simulink model "MASS"  (R2018b)
settings: Solver=VariableStepAuto  StartTime=0.0  StopTime=10.0  RelTol=1e-3
values from neighbouring files (symbols this model uses):
  B = magic(4)    [exp13003.m]    (also in lab13003.m; lab1a3003.m = 2.5; lab2a3003.m = 2.5)
  F = 8    [lab1a3003.m]    (also in lab2a3003.m)
  K = 16    [lab1a3003.m]    (also in lab2a3003.m)
  M = 2    [lab1a3003.m]    (also in lab2a3003.m)
  x0 = 4    [lab1a3003.m]    (also in lab2a3003.m)
settings Model: Creator=student  LastModifiedBy=student

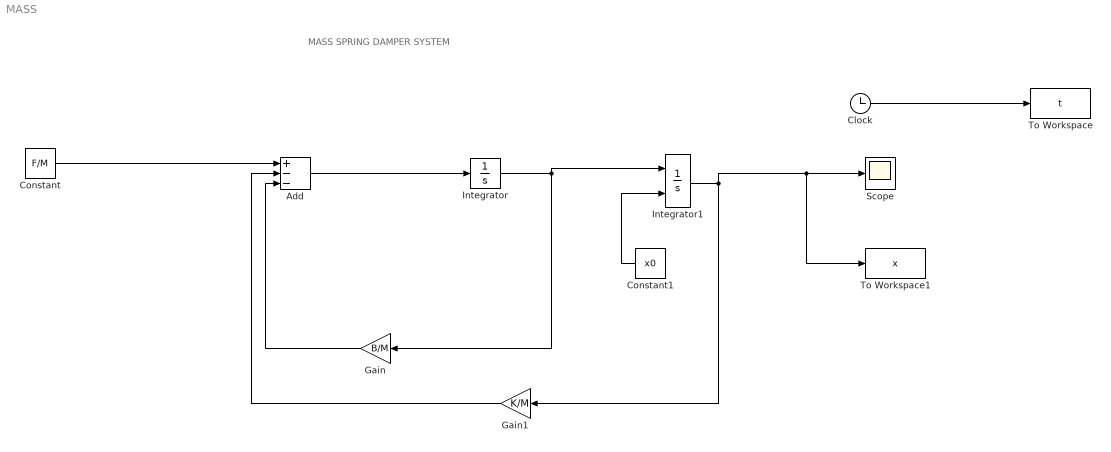
== system MASS ==
  note: MASS SPRING DAMPER SYSTEM
  Add : Sum  Inputs=+--
  Clock : Clock
  Constant : Constant  Value=F/M
  Constant1 : Constant  Value=x0
  Gain : Gain  Gain=B/M
  Gain1 : Gain  Gain=K/M
  Integrator : Integrator
  Integrator1 : Integrator  InitialConditionSource=external
  Scope : Scope
  To Workspace : ToWorkspace  VariableName=t  SampleTime=-1
  To Workspace1 : ToWorkspace  VariableName=x  SampleTime=-1
  wires:
  Constant/1 -> Add/1
  Add/1 -> Integrator/1
  Integrator/1 -> Gain/1, Integrator1/1
  Integrator1/1 -> Gain1/1, To Workspace1/1, Scope/1
  Gain/1 -> Add/3
  Gain1/1 -> Add/2
  Clock/1 -> To Workspace/1
  Constant1/1 -> Integrator1/2
